simulink model "PVPanel"  (R2021b)
settings: Solver=FixedStepDiscrete  StartTime=0.0  StopTime=inf  RelTol=1e-3
PreLoadFcn:
  | %
  | Fc=3780;                          % PWM Carrier frequency (Hz)
  | Ts_Power=1/Fc/200;         % Simscape Power Systems sample time (s)
  | Ts_Control=20*Ts_Power;  % Inverter Control system sample time (s)
InitFcn:
  | %
  | Fc=3780;                          % PWM Carrier frequency (Hz)
  | Ts_Power=1/Fc/200;         % Simscape Power Systems sample time (s)
  | Ts_Control=20*Ts_Power;  % Inverter Control system sample time (s)
undefined symbols (not defined in the file): Acid, Lead
libraries: spsGroundLib x18, spsVoltageMeasurementLib x18, spsCurrentMeasurementLib x12, spsSeriesRLCBranchLib x10, spsParallelRLCBranchLib x6, spsBreakerLib x6, spsDiodeLib x6, spsBoostConverterLib x4, spsBatteryLib x2, spsPVArrayLib x2, spspowerguiLib x1
settings Model: Creator=MathWorks  LastModifiedBy=masangofi
settings SolverCC: AlgebraicLoopSolver=TrustRegion
settings DataIOCC: SaveFormat=Structure  SignalLoggingSaveFormat=ModelDataLogs  SaveOutput=off  SignalLogging=off  DSMLogging=off  SaveTime=off  ReturnWorkspaceOutputs=off
settings OptimizationCC: ExpressionDepthLimit=2147483647  LifeSpan=inf
settings DebuggingCC: UnderspecifiedInitializationDetection=Classic  MergeDetectMultiDrivingBlocksExec=none  SolverPrmCheckMsg=warning  FcnCallInpInsideContextMsg=warning  AllowSymbolicDim=off  StateNameClashWarn=warning  SFUnexpectedBacktrackingDiag=warning  SFNoUnconditionalDefaultTransitionDiag=warning  SFExecutionAtInitializationDiag=none  SFMachineParentedDataDiag=warning  ArithmeticOperatorsInVariantConditions=warning
settings HardwareCC: ProdBitPerPointer=32  ProdBitPerSizeT=32  ProdBitPerPtrDiffT=32  ProdLargestAtomicFloat=None  ProdIntDivRoundTo=Undefined  ProdEndianess=Unspecified  ProdWordSize=32  ProdHWDeviceType=32-bit Generic
settings ModelReferenceCC: PropagateSignalLabelsOutOfModel=off
settings SFSimCC: SimUseLocalCustomCode=off  CustomCodeUndefinedFunction=UseInterfaceOnly
settings RTWCC: RTWUseLocalCustomCode=off
settings CodeAppCC: StateflowObjectComments=on
settings GRTTargetCC: TargetLangStandard=C89/C90 (ANSI)  CombineOutputUpdateFcns=off  GRTInterface=on
settings ConfigComp: CovMetricSettings=dw  CovSaveCumulativeToWorkspaceVar=on  CovSaveSingleToWorkspaceVar=on  CovExternalEMLEnable=off  CovSFcnEnable=off
settings SimscapeCC: SimscapeNormalizeSystem=off

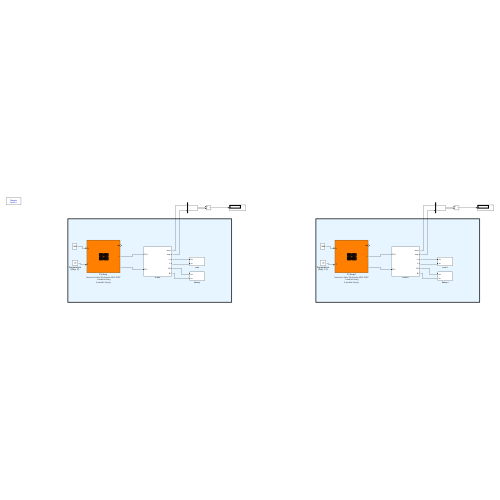
[thumbnail: Simulink's stored preview of the top-level diagram]
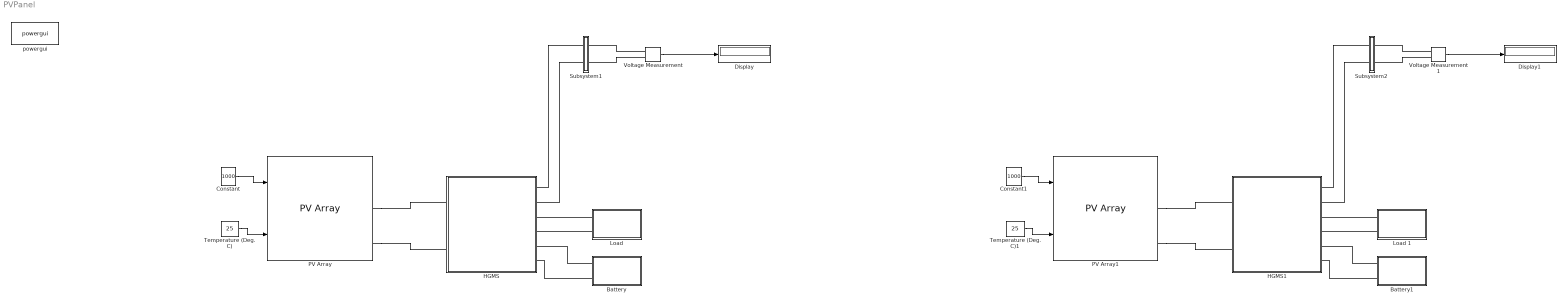
== system PVPanel ==
  Battery : Subsystem
  Battery1 : Subsystem
  Constant : Constant  Value=1000
  Constant1 : Constant  Value=1000
  Display : Display
  Display1 : Display
  HGMS : Subsystem
  HGMS1 : Subsystem
  "Load " : Subsystem
  Load 1 : Subsystem
  PV Array : spsPVArrayLib/PV Array  Npar=5  Nser=1  PlotType=one module @ 25 deg.C & specified irradiances  S_vec=[160 80 40 20 10 ]  Temp_C_vec=[ 4 ]  ModuleName=American Solar Wholesale ASW-220P  PlotWhenSelected=off  Pm=219.765  Ncell=60  Voc=36.24  Isc=7.77  Vm=29.9  Im=7.35  beta_Voc_pc=-0.33  alpha_Isc_pc=0.05  beta_Voc=-0.11959  alpha_Isc=0.003885  IL=7.8511  I0=8.7896e-11  nI=0.9332  Rsh=197.4106  Rs=0.27009  RobustModel=off  RobustCellTemperature=313.3991  BAL=on  Tc=1e-6  Tfilter=5e-5
      settings: AttributesFormatString=|
      | %<ModuleName>
      | %<Nser>-module string
      | %<Npar> parallel strings
  PV Array1 : spsPVArrayLib/PV Array  Npar=5  Nser=1  PlotType=one module @ 25 deg.C & specified irradiances  S_vec=[160 80 40 20 10 ]  Temp_C_vec=[ 4 ]  ModuleName=American Solar Wholesale ASW-220P  PlotWhenSelected=off  Pm=219.765  Ncell=60  Voc=36.24  Isc=7.77  Vm=29.9  Im=7.35  beta_Voc_pc=-0.33  alpha_Isc_pc=0.05  beta_Voc=-0.11959  alpha_Isc=0.003885  IL=7.8511  I0=8.7896e-11  nI=0.9332  Rsh=197.4106  Rs=0.27009  RobustModel=off  RobustCellTemperature=313.3991  BAL=on  Tc=1e-6  Tfilter=5e-5
      settings: AttributesFormatString=|
      | %<ModuleName>
      | %<Nser>-module string
      | %<Npar> parallel strings
  Subsystem1 : Subsystem
  Subsystem2 : Subsystem
  Temperature (Deg. C) : Constant  Value=25
  Temperature (Deg. C)1 : Constant  Value=25
  Voltage Measurement : spsVoltageMeasurementLib/Voltage Measurement  PhasorSimulation=off  OutputType=Complex  PSBequivalent=0
  Voltage Measurement1 : spsVoltageMeasurementLib/Voltage Measurement  PhasorSimulation=off  OutputType=Complex  PSBequivalent=0
  powergui : spspowerguiLib/powergui  Priority=1  SimulationMode=Discrete  SampleTime=50e-6  frequency=60  Iterations=50  frequencyindice=0  Pbase=100e6  ErrMax=1e-4  UnitsV=kV  UnitsW=MW  buscounter=0  FunctionMessages=off  echomessages=off  EnableUseOfTLC=off  CurrentSourceSwitches=off  DisableSnubberDevices=off  DisableRonSwitches=off  DisableVfSwitches=off  DisplayEquations=off  AutomaticDiscreteSolvers=off  SolverType=Tustin/Backward Euler (TBE)  Interpol=off  ExternalGateDelay=off  methode=off  Ts=100  x0status=blocks  SPID=on  SwTol=0  HookPort=off  NonlinearTolerance=1e-4  nMaxIteration=100  ContinueOnMaxIteration=off  RestoreLinks=warning  ResistiveCurrentMeasurement=off  Frange=[0:2:500]  Ylog=off  Xlog=on  ShowGrid=off  save=off  variable=ZData  structure=0  ZoomFFT=off  StartTime=0.0  cycles=1  DisplayStyle=1  fundamental=60  FreqAxis=off  MaxFrequency=1000  frequencyindicesteady=1  RmsSteady=1  display=off
  wires:
  Temperature (Deg. C)/1 -> PV Array/2
  Constant/1 -> PV Array/1
  Voltage Measurement/1 -> Display/1
  Voltage Measurement1/1 -> Display1/1
  Constant1/1 -> PV Array1/1
  Temperature (Deg. C)1/1 -> PV Array1/2
  connections:
  "Load "/LConn2 -- HGMS/RConn4
  Subsystem1/LConn2 -- HGMS/RConn2
  Subsystem1/LConn1 -- HGMS/RConn1
  Voltage Measurement/LConn1 -- Subsystem1/RConn1
  Voltage Measurement/LConn2 -- Subsystem1/RConn2
  Battery/LConn2 -- HGMS/RConn6
  Battery/LConn1 -- HGMS/RConn5
  "Load "/LConn1 -- HGMS/RConn3
  PV Array/RConn2 -- HGMS/LConn2
  PV Array/RConn1 -- HGMS/LConn1
  Voltage Measurement1/LConn1 -- Subsystem2/RConn1
  Load 1/LConn1 -- HGMS1/RConn3
  Load 1/LConn2 -- HGMS1/RConn4
  Subsystem2/LConn2 -- HGMS1/RConn2
  Subsystem2/LConn1 -- HGMS1/RConn1
  Battery1/LConn2 -- HGMS1/RConn6
  Battery1/LConn1 -- HGMS1/RConn5
  PV Array1/RConn1 -- HGMS1/LConn1
  PV Array1/RConn2 -- HGMS1/LConn2
  Voltage Measurement1/LConn2 -- Subsystem2/RConn2

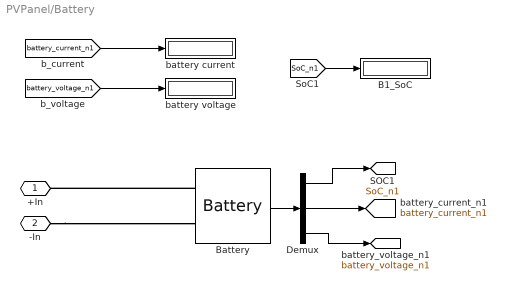
== system PVPanel/Battery ==
  B1_SoC : Display
  Battery : spsBatteryLib/Battery  BatType=Lead-Acid  ShowTempParam=off  ThermalPreset=no  ShowAgeParam=off  NomV=48  NomQ=70  SOC=70  Batt_Tr=1  PresetModel=on  MaxQ=72.9167  MinV=36  FullV=52.2632  Dis_rate=14  R=0.0068571  Normal_OP=21.7194  expZone="[48.8684     0.233333]"  current=[6.5 13 32.5]  Units=Time  Tci=20  NomT=20  T2=-30  MaxQ2=4.8  FullV2=7.1  Normal_OP2=5.655  expZone2="[6.58           1]"  Rca=0.6  ti=2000  Dp=0  Neq0=0  Tsim=1e6  Ta1=25  Qeol=5.4*0.9  Reol=0.013333*1.2  Char_age=[2.3478, 3]  Dis_age=[2.3478, 10]  N1=1500  N2=10500  N3=1000  N4=1400  Ta2=45  N5=950
  Demux : Demux  Outputs=3
  battery current : Display
  battery voltage : Display
  +In : PMIOPort  Side=Left
  -In : PMIOPort  Port=2  Side=Left
  tag scope: SoC_n1=global, battery_current_n1=global, battery_voltage_n1=global
  wires:
  Battery/1 -> Demux/1
  Demux/1 -> [SoC_n1]
  Demux/3 -> [battery_voltage_n1]
  Demux/2 -> [battery_current_n1]
  [SoC_n1] -> B1_SoC/1
  [battery_current_n1] -> battery current/1
  [battery_voltage_n1] -> battery voltage/1
  connections:
  -In/RConn1 -- Battery/LConn2
  Battery/LConn1 -- +In/RConn1

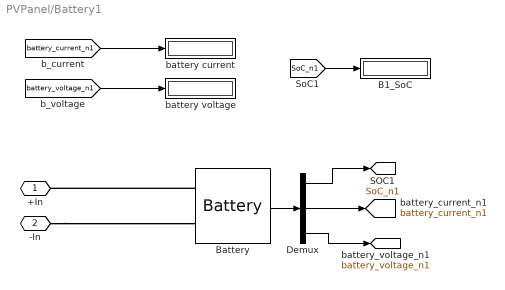
== system PVPanel/Battery1 ==
  B1_SoC : Display
  Battery : spsBatteryLib/Battery  BatType=Lead-Acid  ShowTempParam=off  ThermalPreset=no  ShowAgeParam=off  NomV=48  NomQ=70  SOC=70  Batt_Tr=1  PresetModel=on  MaxQ=72.9167  MinV=36  FullV=52.2632  Dis_rate=14  R=0.0068571  Normal_OP=21.7194  expZone="[48.8684     0.233333]"  current=[6.5 13 32.5]  Units=Time  Tci=20  NomT=20  T2=-30  MaxQ2=4.8  FullV2=7.1  Normal_OP2=5.655  expZone2="[6.58           1]"  Rca=0.6  ti=2000  Dp=0  Neq0=0  Tsim=1e6  Ta1=25  Qeol=5.4*0.9  Reol=0.013333*1.2  Char_age=[2.3478, 3]  Dis_age=[2.3478, 10]  N1=1500  N2=10500  N3=1000  N4=1400  Ta2=45  N5=950
  Demux : Demux  Outputs=3
  battery current : Display
  battery voltage : Display
  +In : PMIOPort  Side=Left
  -In : PMIOPort  Port=2  Side=Left
  tag scope: SoC_n1=global, battery_current_n1=global, battery_voltage_n1=global
  wires:
  Battery/1 -> Demux/1
  Demux/1 -> [SoC_n1]
  Demux/3 -> [battery_voltage_n1]
  Demux/2 -> [battery_current_n1]
  [SoC_n1] -> B1_SoC/1
  [battery_current_n1] -> battery current/1
  [battery_voltage_n1] -> battery voltage/1
  connections:
  -In/RConn1 -- Battery/LConn2
  Battery/LConn1 -- +In/RConn1

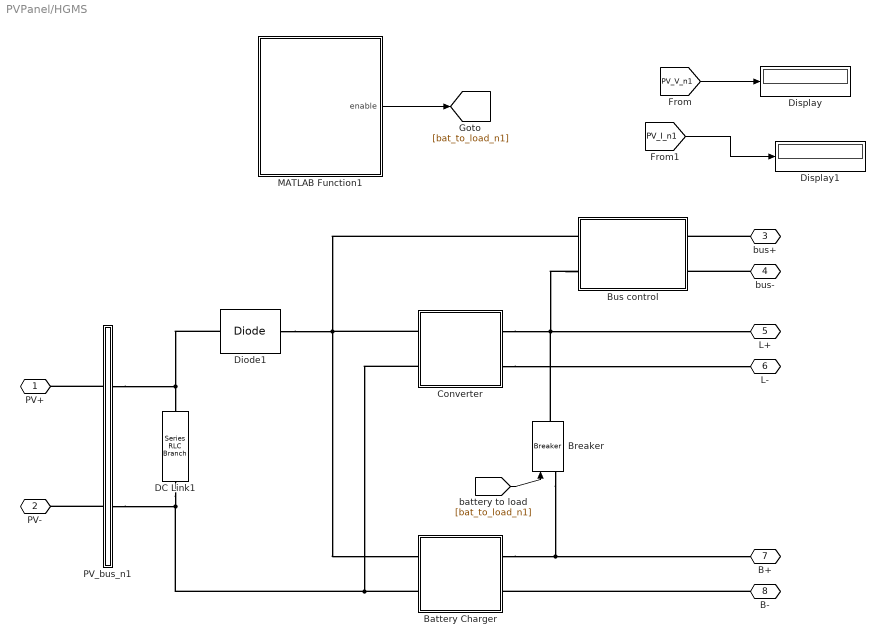
== system PVPanel/HGMS ==
  Battery Charger : Subsystem
  Breaker : spsBreakerLib/Breaker  InitialState=0  SwitchingTimes="[1/60  5/60]"  External=on  BreakerResistance=0.01  SnubberResistance=1e6  SnubberCapacitance=inf  Measurements=None  MoreParameters=on  NoBreakLoop=off
      settings: SourceProductBaseCode=PS
  Bus control : Subsystem
  Converter : Subsystem
  DC Link1 : spsSeriesRLCBranchLib/Series RLC Branch  LConnTagsString=__new0  RConnTagsString=__new0  BranchType=C  Resistance=1.0  Inductance=1.0  SetiL0=off  InitialCurrent=0  Capacitance=1000e-6  Setx0=off  InitialVoltage=48  Measurements=None
  Diode1 : spsDiodeLib/Diode  Ron=0.001  Lon=0  Vf=0.8  IC=0  UseSnubber=0  Rs=inf  Cs=250e-9  Measurements=off
  Display : Display
  Display1 : Display
  MATLAB Function1 : MATLAB Function  TreatAsAtomicUnit=on
  PV_bus_n1 : Subsystem
  PV+ : PMIOPort  Side=Left
  PV- : PMIOPort  Port=2  Side=Left
  bus+ : PMIOPort  Port=3  Side=Right
  bus- : PMIOPort  Port=4  Side=Right
  L+ : PMIOPort  Port=5  Side=Right
  L- : PMIOPort  Port=6  Side=Right
  B+ : PMIOPort  Port=7  Side=Right
  B- : PMIOPort  Port=8  Side=Right
  wires:
  MATLAB Function1/1(enable) -> [bat_to_load_n1]
  [bat_to_load_n1] -> Breaker/1
  [PV_V_n1] -> Display/1
  [PV_I_n1] -> Display1/1
  connections:
  Battery Charger/LConn2 -- Converter/LConn2 -- PV_bus_n1/RConn2 -- DC Link1/RConn1
  Converter/RConn1 -- Bus control/LConn2 -- Breaker/RConn1 -- L+/RConn1
  Converter/RConn2 -- L-/RConn1
  bus-/RConn1 -- Bus control/RConn2
  bus+/RConn1 -- Bus control/RConn1
  Battery Charger/RConn1 -- Breaker/LConn1 -- B+/RConn1
  B-/RConn1 -- Battery Charger/RConn2
  Diode1/RConn1 -- Bus control/LConn1 -- Converter/LConn1 -- Battery Charger/LConn1
  Diode1/LConn1 -- PV_bus_n1/RConn1 -- DC Link1/LConn1
  PV_bus_n1/LConn1 -- PV+/RConn1
  PV_bus_n1/LConn2 -- PV-/RConn1

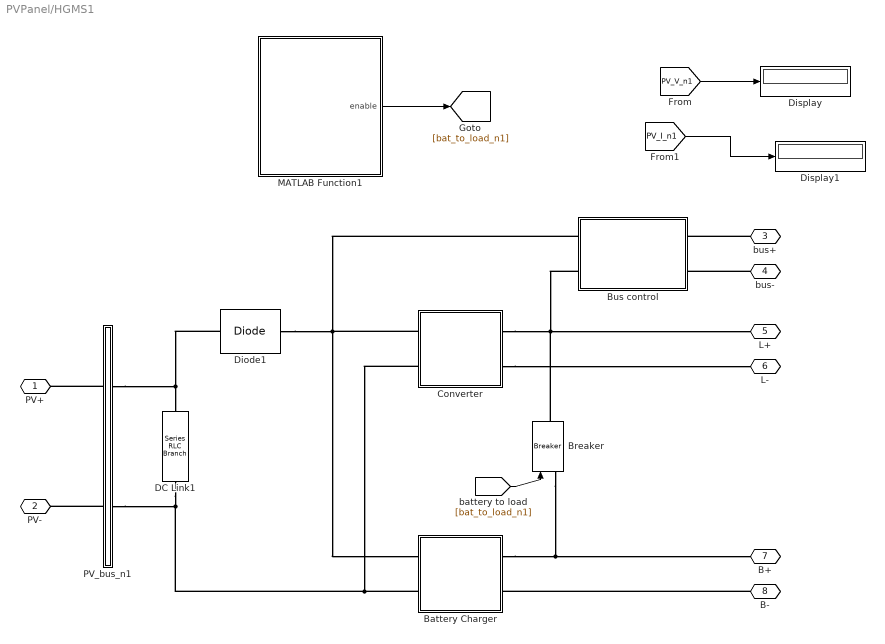
== system PVPanel/HGMS1 ==
  Battery Charger : Subsystem
  Breaker : spsBreakerLib/Breaker  InitialState=0  SwitchingTimes="[1/60  5/60]"  External=on  BreakerResistance=0.01  SnubberResistance=1e6  SnubberCapacitance=inf  Measurements=None  MoreParameters=on  NoBreakLoop=off
      settings: SourceProductBaseCode=PS
  Bus control : Subsystem
  Converter : Subsystem
  DC Link1 : spsSeriesRLCBranchLib/Series RLC Branch  LConnTagsString=__new0  RConnTagsString=__new0  BranchType=C  Resistance=1.0  Inductance=1.0  SetiL0=off  InitialCurrent=0  Capacitance=1000e-6  Setx0=off  InitialVoltage=48  Measurements=None
  Diode1 : spsDiodeLib/Diode  Ron=0.001  Lon=0  Vf=0.8  IC=0  UseSnubber=0  Rs=inf  Cs=250e-9  Measurements=off
  Display : Display
  Display1 : Display
  MATLAB Function1 : MATLAB Function  TreatAsAtomicUnit=on
  PV_bus_n1 : Subsystem
  PV+ : PMIOPort  Side=Left
  PV- : PMIOPort  Port=2  Side=Left
  bus+ : PMIOPort  Port=3  Side=Right
  bus- : PMIOPort  Port=4  Side=Right
  L+ : PMIOPort  Port=5  Side=Right
  L- : PMIOPort  Port=6  Side=Right
  B+ : PMIOPort  Port=7  Side=Right
  B- : PMIOPort  Port=8  Side=Right
  wires:
  MATLAB Function1/1(enable) -> [bat_to_load_n1]
  [bat_to_load_n1] -> Breaker/1
  [PV_V_n1] -> Display/1
  [PV_I_n1] -> Display1/1
  connections:
  Battery Charger/LConn2 -- PV_bus_n1/RConn2 -- DC Link1/RConn1 -- Converter/LConn2
  Converter/RConn1 -- Breaker/RConn1 -- L+/RConn1 -- Bus control/LConn2
  Converter/RConn2 -- L-/RConn1
  bus-/RConn1 -- Bus control/RConn2
  bus+/RConn1 -- Bus control/RConn1
  Battery Charger/RConn1 -- Breaker/LConn1 -- B+/RConn1
  B-/RConn1 -- Battery Charger/RConn2
  Converter/LConn1 -- Battery Charger/LConn1 -- Diode1/RConn1 -- Bus control/LConn1
  Diode1/LConn1 -- DC Link1/LConn1 -- PV_bus_n1/RConn1
  PV_bus_n1/LConn1 -- PV+/RConn1
  PV_bus_n1/LConn2 -- PV-/RConn1

== system PVPanel/Load  ==
  Parallel RLC Branch : spsParallelRLCBranchLib/Parallel RLC Branch  LConnTagsString=a  RConnTagsString=__new0  BranchType=R  Resistance=10000  Inductance=1e-3  SetiL0=off  InitialCurrent=0  Capacitance=1e-6  Setx0=off  InitialVoltage=0  Measurements=None
  +In : PMIOPort  Side=Left
  -In : PMIOPort  Port=2  Side=Left
  connections:
  Parallel RLC Branch/LConn1 -- +In/RConn1
  -In/RConn1 -- Parallel RLC Branch/RConn1

== system PVPanel/Load 1 ==
  Parallel RLC Branch : spsParallelRLCBranchLib/Parallel RLC Branch  LConnTagsString=a  RConnTagsString=__new0  BranchType=R  Resistance=10000  Inductance=1e-3  SetiL0=off  InitialCurrent=0  Capacitance=1e-6  Setx0=off  InitialVoltage=0  Measurements=None
  +In : PMIOPort  Side=Left
  -In : PMIOPort  Port=2  Side=Left
  connections:
  Parallel RLC Branch/LConn1 -- +In/RConn1
  -In/RConn1 -- Parallel RLC Branch/RConn1

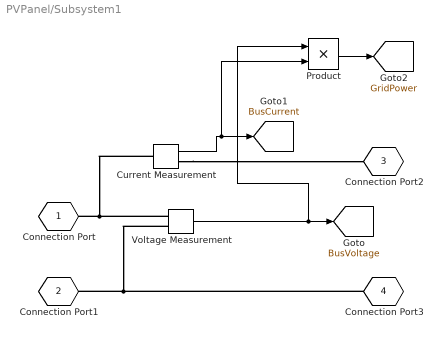
== system PVPanel/Subsystem1 ==
  Current Measurement : spsCurrentMeasurementLib/Current Measurement  PhasorSimulation=off  OutputType=Complex  PSBequivalent=0
  Product : Product
  Voltage Measurement : spsVoltageMeasurementLib/Voltage Measurement  PhasorSimulation=off  OutputType=Complex  PSBequivalent=0
  Connection Port : PMIOPort  Tag=PMCPort  Side=Left
  Connection Port1 : PMIOPort  Tag=PMCPort  Port=2  Side=Left
  Connection Port2 : PMIOPort  Tag=PMCPort  Port=3  Side=Right
  Connection Port3 : PMIOPort  Tag=PMCPort  Port=4  Side=Right
  tag scope: BusCurrent=global, BusVoltage=global, GridPower=global
  wires:
  Current Measurement/1 -> Product/2, [BusCurrent]
  Voltage Measurement/1 -> Product/1, [BusVoltage]
  Product/1 -> [GridPower]
  connections:
  Current Measurement/LConn1 -- Voltage Measurement/LConn1 -- Connection Port/RConn1
  Current Measurement/RConn1 -- Connection Port2/RConn1
  Voltage Measurement/LConn2 -- Connection Port3/RConn1 -- Connection Port1/RConn1

== system PVPanel/Subsystem2 ==
  Current Measurement : spsCurrentMeasurementLib/Current Measurement  PhasorSimulation=off  OutputType=Complex  PSBequivalent=0
  Product : Product
  Voltage Measurement : spsVoltageMeasurementLib/Voltage Measurement  PhasorSimulation=off  OutputType=Complex  PSBequivalent=0
  Connection Port : PMIOPort  Tag=PMCPort  Side=Left
  Connection Port1 : PMIOPort  Tag=PMCPort  Port=2  Side=Left
  Connection Port2 : PMIOPort  Tag=PMCPort  Port=3  Side=Right
  Connection Port3 : PMIOPort  Tag=PMCPort  Port=4  Side=Right
  tag scope: BusCurrent=global, BusVoltage=global, GridPower=global
  wires:
  Current Measurement/1 -> Product/2, [BusCurrent]
  Voltage Measurement/1 -> Product/1, [BusVoltage]
  Product/1 -> [GridPower]
  connections:
  Current Measurement/LConn1 -- Voltage Measurement/LConn1 -- Connection Port/RConn1
  Current Measurement/RConn1 -- Connection Port2/RConn1
  Voltage Measurement/LConn2 -- Connection Port3/RConn1 -- Connection Port1/RConn1

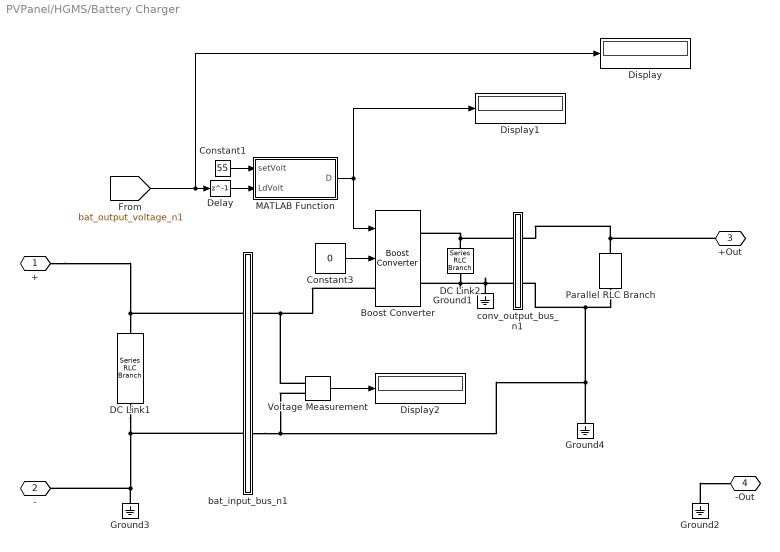
== system PVPanel/HGMS/Battery Charger ==
  Boost Converter : spsBoostConverterLib/Boost Converter  ModelType=Average model (D-controlled)  Ron=1e-6  Rs=1e6  Cs=inf  Vforward=[0,0]  Ron_Diode=1e-3  Rs_Diode=1e6  Cs_Diode=inf  Vf_Diode=1e-3  Rs_CurrentSource=1e6
      settings: SourceProductBaseCode=PS
  Constant1 : Constant  Value=55  OutDataTypeStr=double
  Constant3 : Constant  Value=0
  DC Link1 : spsSeriesRLCBranchLib/Series RLC Branch  LConnTagsString=__new0  RConnTagsString=__new0  BranchType=C  Resistance=1.0  Inductance=1.0  SetiL0=off  InitialCurrent=0  Capacitance=1000e-6  Setx0=off  InitialVoltage=0  Measurements=None
  DC Link2 : spsSeriesRLCBranchLib/Series RLC Branch  LConnTagsString=__new0  RConnTagsString=__new0  BranchType=C  Resistance=1.0  Inductance=1.0  SetiL0=off  InitialCurrent=0  Capacitance=100e-6  Setx0=off  InitialVoltage=0  Measurements=None
  Delay : Delay  DelayLength=1  InitialCondition=0
  Display : Display
  Display1 : Display
  Display2 : Display
  Ground{1..4} (4 alike) : spsGroundLib/Ground  LConnTagsString=a
  MATLAB Function : MATLAB Function  TreatAsAtomicUnit=on
  Parallel RLC Branch : spsParallelRLCBranchLib/Parallel RLC Branch  LConnTagsString=a  RConnTagsString=__new0  BranchType=R  Resistance=10e3  Inductance=1e-3  SetiL0=off  InitialCurrent=0  Capacitance=1e-6  Setx0=off  InitialVoltage=0  Measurements=None
  Voltage Measurement : spsVoltageMeasurementLib/Voltage Measurement  PhasorSimulation=off  OutputType=Complex  PSBequivalent=0
  bat_input_bus_n1 : Subsystem
  conv_output_bus_n1 : Subsystem
  + : PMIOPort  Side=Left
  - : PMIOPort  Port=2  Side=Left
  +Out : PMIOPort  Port=3  Side=Right
  -Out : PMIOPort  Port=4  Side=Right
  wires:
  Delay/1 -> MATLAB Function/2(LdVolt)
  [bat_output_voltage_n1] -> Display/1, Delay/1
  Constant3/1 -> Boost Converter/2
  Constant1/1 -> MATLAB Function/1(setVolt)
  MATLAB Function/1(D) -> Boost Converter/1, Display1/1
  Voltage Measurement/1 -> Display2/1
  connections:
  +/RConn1 -- DC Link1/LConn1 -- bat_input_bus_n1/LConn1
  DC Link1/RConn1 -- Ground3/LConn1 -- -/RConn1 -- bat_input_bus_n1/LConn2
  Boost Converter/RConn2 -- DC Link2/RConn1 -- conv_output_bus_n1/LConn2 -- Ground1/LConn1
  DC Link2/LConn1 -- Boost Converter/RConn1 -- conv_output_bus_n1/LConn1
  Ground4/LConn1 -- Voltage Measurement/LConn2 -- bat_input_bus_n1/RConn2 -- conv_output_bus_n1/RConn2 -- Parallel RLC Branch/RConn1
  Parallel RLC Branch/LConn1 -- conv_output_bus_n1/RConn1 -- +Out/RConn1
  Boost Converter/LConn1 -- Voltage Measurement/LConn1 -- bat_input_bus_n1/RConn1
  Ground2/LConn1 -- -Out/RConn1

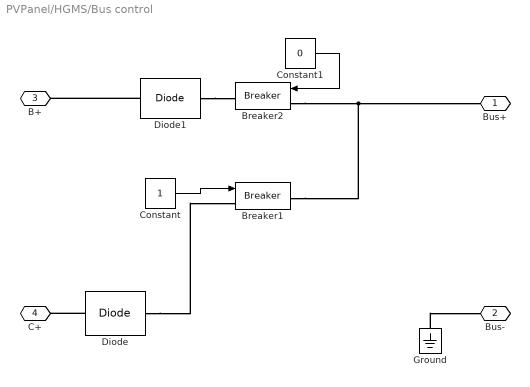
== system PVPanel/HGMS/Bus control ==
  Breaker1 : spsBreakerLib/Breaker  InitialState=0  SwitchingTimes="[1/60  5/60]"  External=on  BreakerResistance=0.01  SnubberResistance=1e6  SnubberCapacitance=inf  Measurements=None  MoreParameters=on  NoBreakLoop=off
      settings: SourceProductBaseCode=PS
  Breaker2 : spsBreakerLib/Breaker  InitialState=0  SwitchingTimes="[1/60  5/60]"  External=on  BreakerResistance=0.01  SnubberResistance=1e6  SnubberCapacitance=inf  Measurements=None  MoreParameters=on  NoBreakLoop=off
      settings: SourceProductBaseCode=PS
  Constant : Constant
  Constant1 : Constant  Value=0
  Diode : spsDiodeLib/Diode  Ron=0.001  Lon=0  Vf=0.8  IC=0  UseSnubber=0  Rs=500  Cs=250e-9  Measurements=off
  Diode1 : spsDiodeLib/Diode  Ron=0.001  Lon=0  Vf=0.8  IC=0  UseSnubber=0  Rs=500  Cs=250e-9  Measurements=off
  Ground : spsGroundLib/Ground  LConnTagsString=a
  Bus+ : PMIOPort  Side=Right
  Bus- : PMIOPort  Port=2  Side=Right
  B+ : PMIOPort  Port=3  Side=Left
  C+ : PMIOPort  Port=4  Side=Left
  wires:
  Constant/1 -> Breaker1/1
  Constant1/1 -> Breaker2/1
  connections:
  Breaker1/RConn1 -- Breaker2/LConn1 -- Bus+/RConn1
  Ground/LConn1 -- Bus-/RConn1
  Diode/LConn1 -- C+/RConn1
  Diode/RConn1 -- Breaker1/LConn1
  Diode1/RConn1 -- B+/RConn1
  Diode1/LConn1 -- Breaker2/RConn1

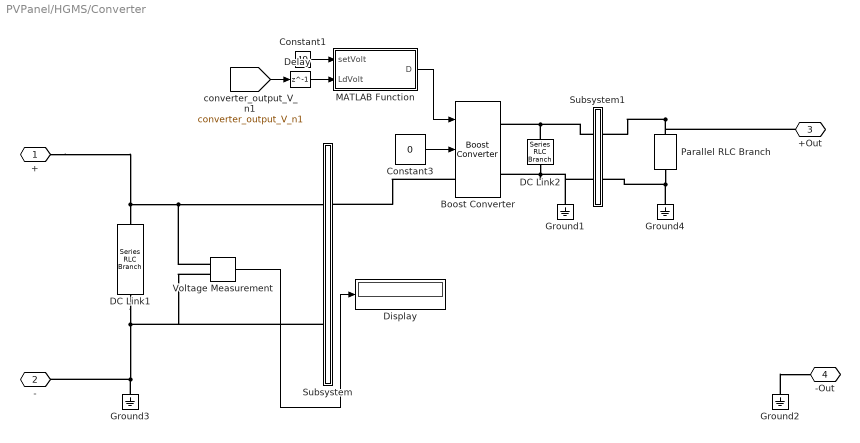
== system PVPanel/HGMS/Converter ==
  Boost Converter : spsBoostConverterLib/Boost Converter  ModelType=Average model (D-controlled)  Ron=1e-6  Rs=1e6  Cs=inf  Vforward=[0,0]  Ron_Diode=1e-3  Rs_Diode=1e6  Cs_Diode=inf  Vf_Diode=1e-3  Rs_CurrentSource=inf
      settings: SourceProductBaseCode=PS
  Constant1 : Constant  Value=49  OutDataTypeStr=double
  Constant3 : Constant  Value=0
  DC Link1 : spsSeriesRLCBranchLib/Series RLC Branch  LConnTagsString=__new0  RConnTagsString=__new0  BranchType=C  Resistance=1.0  Inductance=1.0  SetiL0=off  InitialCurrent=0  Capacitance=1000e-6  Setx0=off  InitialVoltage=0  Measurements=None
  DC Link2 : spsSeriesRLCBranchLib/Series RLC Branch  LConnTagsString=__new0  RConnTagsString=__new0  BranchType=C  Resistance=1.0  Inductance=1.0  SetiL0=off  InitialCurrent=0  Capacitance=100e-6  Setx0=off  InitialVoltage=0  Measurements=None
  Delay : Delay  DelayLength=1  InitialCondition=0
  Display : Display
  Ground{1..4} (4 alike) : spsGroundLib/Ground  LConnTagsString=a
  MATLAB Function : MATLAB Function  TreatAsAtomicUnit=on
  Parallel RLC Branch : spsParallelRLCBranchLib/Parallel RLC Branch  LConnTagsString=a  RConnTagsString=__new0  BranchType=R  Resistance=10e3  Inductance=1e-3  SetiL0=off  InitialCurrent=0  Capacitance=1e-6  Setx0=off  InitialVoltage=0  Measurements=None
  Subsystem : Subsystem
  Subsystem1 : Subsystem
  Voltage Measurement : spsVoltageMeasurementLib/Voltage Measurement  PhasorSimulation=off  OutputType=Complex  PSBequivalent=0
  + : PMIOPort  Side=Left
  - : PMIOPort  Port=2  Side=Left
  +Out : PMIOPort  Port=3  Side=Right
  -Out : PMIOPort  Port=4  Side=Right
  wires:
  Delay/1 -> MATLAB Function/2(LdVolt)
  [converter_output_V_n1] -> Delay/1
  Constant3/1 -> Boost Converter/2
  Constant1/1 -> MATLAB Function/1(setVolt)
  MATLAB Function/1(D) -> Boost Converter/1
  Voltage Measurement/1 -> Display/1
  connections:
  +/RConn1 -- Voltage Measurement/LConn1 -- Subsystem/LConn1 -- DC Link1/LConn1
  DC Link1/RConn1 -- Voltage Measurement/LConn2 -- Subsystem/LConn2 -- Ground3/LConn1 -- -/RConn1
  DC Link2/RConn1 -- Subsystem1/LConn2 -- Ground1/LConn1 -- Boost Converter/RConn2
  DC Link2/LConn1 -- Subsystem1/LConn1 -- Boost Converter/RConn1
  Parallel RLC Branch/RConn1 -- Subsystem1/RConn2 -- Ground4/LConn1
  Boost Converter/LConn1 -- Subsystem/RConn1
  Ground2/LConn1 -- -Out/RConn1
  Parallel RLC Branch/LConn1 -- Subsystem1/RConn1 -- +Out/RConn1

== system PVPanel/HGMS/PV_bus_n1 ==
  Current Measurement : spsCurrentMeasurementLib/Current Measurement  PhasorSimulation=off  OutputType=Complex  PSBequivalent=0
  Voltage Measurement : spsVoltageMeasurementLib/Voltage Measurement  PhasorSimulation=off  OutputType=Complex  PSBequivalent=0
  Connection Port : PMIOPort  Tag=PMCPort  Side=Left
  Connection Port1 : PMIOPort  Tag=PMCPort  Port=2  Side=Left
  Connection Port2 : PMIOPort  Tag=PMCPort  Port=3  Side=Right
  Connection Port3 : PMIOPort  Tag=PMCPort  Port=4  Side=Right
  tag scope: PV_I_n1=global, PV_V_n1=global
  wires:
  Current Measurement/1 -> [PV_I_n1]
  Voltage Measurement/1 -> [PV_V_n1]
  connections:
  Current Measurement/LConn1 -- Voltage Measurement/LConn1 -- Connection Port/RConn1
  Current Measurement/RConn1 -- Connection Port2/RConn1
  Voltage Measurement/LConn2 -- Connection Port3/RConn1 -- Connection Port1/RConn1

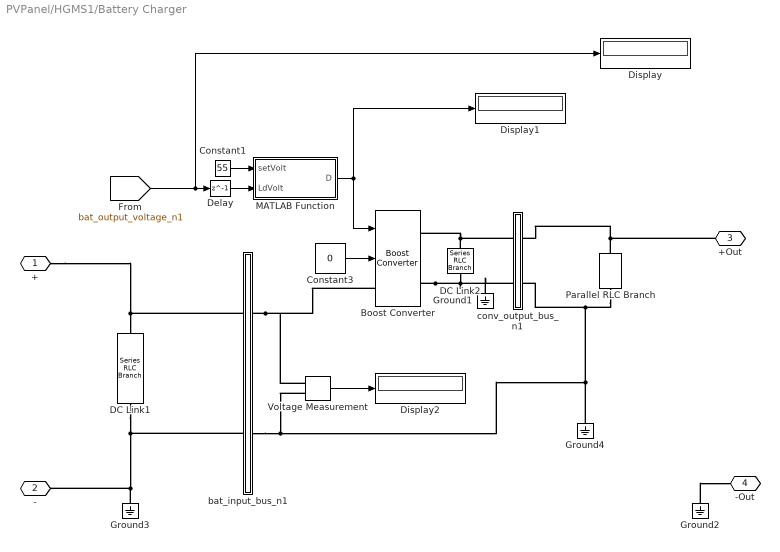
== system PVPanel/HGMS1/Battery Charger ==
  Boost Converter : spsBoostConverterLib/Boost Converter  ModelType=Average model (D-controlled)  Ron=1e-6  Rs=1e6  Cs=inf  Vforward=[0,0]  Ron_Diode=1e-3  Rs_Diode=1e6  Cs_Diode=inf  Vf_Diode=1e-3  Rs_CurrentSource=1e6
      settings: SourceProductBaseCode=PS
  Constant1 : Constant  Value=55  OutDataTypeStr=double
  Constant3 : Constant  Value=0
  DC Link1 : spsSeriesRLCBranchLib/Series RLC Branch  LConnTagsString=__new0  RConnTagsString=__new0  BranchType=C  Resistance=1.0  Inductance=1.0  SetiL0=off  InitialCurrent=0  Capacitance=1000e-6  Setx0=off  InitialVoltage=0  Measurements=None
  DC Link2 : spsSeriesRLCBranchLib/Series RLC Branch  LConnTagsString=__new0  RConnTagsString=__new0  BranchType=C  Resistance=1.0  Inductance=1.0  SetiL0=off  InitialCurrent=0  Capacitance=100e-6  Setx0=off  InitialVoltage=0  Measurements=None
  Delay : Delay  DelayLength=1  InitialCondition=0
  Display : Display
  Display1 : Display
  Display2 : Display
  Ground{1..4} (4 alike) : spsGroundLib/Ground  LConnTagsString=a
  MATLAB Function : MATLAB Function  TreatAsAtomicUnit=on
  Parallel RLC Branch : spsParallelRLCBranchLib/Parallel RLC Branch  LConnTagsString=a  RConnTagsString=__new0  BranchType=R  Resistance=10e3  Inductance=1e-3  SetiL0=off  InitialCurrent=0  Capacitance=1e-6  Setx0=off  InitialVoltage=0  Measurements=None
  Voltage Measurement : spsVoltageMeasurementLib/Voltage Measurement  PhasorSimulation=off  OutputType=Complex  PSBequivalent=0
  bat_input_bus_n1 : Subsystem
  conv_output_bus_n1 : Subsystem
  + : PMIOPort  Side=Left
  - : PMIOPort  Port=2  Side=Left
  +Out : PMIOPort  Port=3  Side=Right
  -Out : PMIOPort  Port=4  Side=Right
  wires:
  Delay/1 -> MATLAB Function/2(LdVolt)
  [bat_output_voltage_n1] -> Display/1, Delay/1
  Constant3/1 -> Boost Converter/2
  Constant1/1 -> MATLAB Function/1(setVolt)
  MATLAB Function/1(D) -> Boost Converter/1, Display1/1
  Voltage Measurement/1 -> Display2/1
  connections:
  +/RConn1 -- DC Link1/LConn1 -- bat_input_bus_n1/LConn1
  DC Link1/RConn1 -- Ground3/LConn1 -- -/RConn1 -- bat_input_bus_n1/LConn2
  Boost Converter/RConn2 -- DC Link2/RConn1 -- conv_output_bus_n1/LConn2 -- Ground1/LConn1
  DC Link2/LConn1 -- Boost Converter/RConn1 -- conv_output_bus_n1/LConn1
  Voltage Measurement/LConn2 -- bat_input_bus_n1/RConn2 -- Ground4/LConn1 -- Parallel RLC Branch/RConn1 -- conv_output_bus_n1/RConn2
  +Out/RConn1 -- Parallel RLC Branch/LConn1 -- conv_output_bus_n1/RConn1
  bat_input_bus_n1/RConn1 -- Boost Converter/LConn1 -- Voltage Measurement/LConn1
  Ground2/LConn1 -- -Out/RConn1

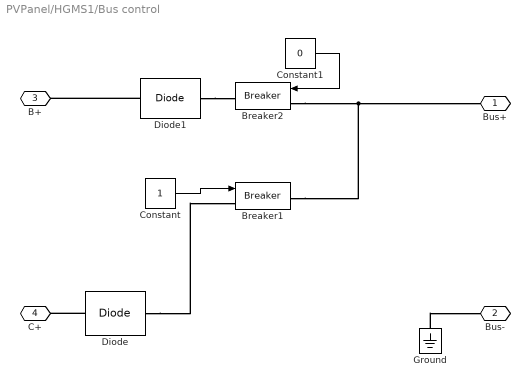
== system PVPanel/HGMS1/Bus control ==
  Breaker1 : spsBreakerLib/Breaker  InitialState=0  SwitchingTimes="[1/60  5/60]"  External=on  BreakerResistance=0.01  SnubberResistance=1e6  SnubberCapacitance=inf  Measurements=None  MoreParameters=on  NoBreakLoop=off
      settings: SourceProductBaseCode=PS
  Breaker2 : spsBreakerLib/Breaker  InitialState=0  SwitchingTimes="[1/60  5/60]"  External=on  BreakerResistance=0.01  SnubberResistance=1e6  SnubberCapacitance=inf  Measurements=None  MoreParameters=on  NoBreakLoop=off
      settings: SourceProductBaseCode=PS
  Constant : Constant
  Constant1 : Constant  Value=0
  Diode : spsDiodeLib/Diode  Ron=0.001  Lon=0  Vf=0.8  IC=0  UseSnubber=0  Rs=500  Cs=250e-9  Measurements=off
  Diode1 : spsDiodeLib/Diode  Ron=0.001  Lon=0  Vf=0.8  IC=0  UseSnubber=0  Rs=500  Cs=250e-9  Measurements=off
  Ground : spsGroundLib/Ground  LConnTagsString=a
  Bus+ : PMIOPort  Side=Right
  Bus- : PMIOPort  Port=2  Side=Right
  B+ : PMIOPort  Port=3  Side=Left
  C+ : PMIOPort  Port=4  Side=Left
  wires:
  Constant/1 -> Breaker1/1
  Constant1/1 -> Breaker2/1
  connections:
  Breaker1/RConn1 -- Bus+/RConn1 -- Breaker2/LConn1
  Ground/LConn1 -- Bus-/RConn1
  Diode/LConn1 -- C+/RConn1
  Diode/RConn1 -- Breaker1/LConn1
  Diode1/RConn1 -- B+/RConn1
  Diode1/LConn1 -- Breaker2/RConn1

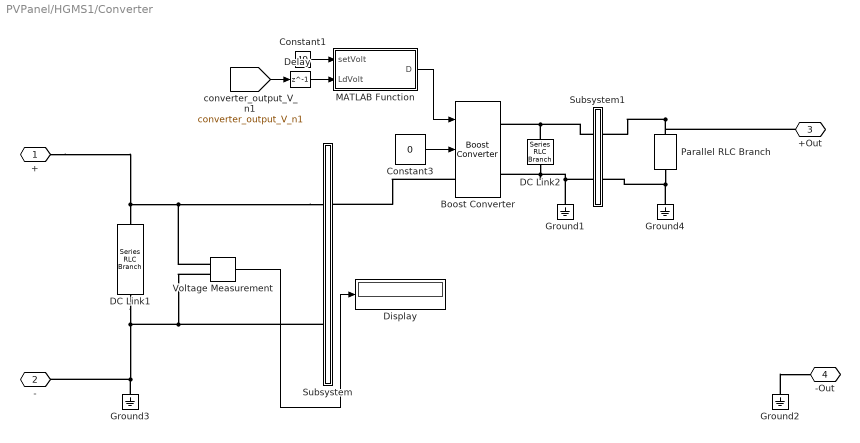
== system PVPanel/HGMS1/Converter ==
  Boost Converter : spsBoostConverterLib/Boost Converter  ModelType=Average model (D-controlled)  Ron=1e-6  Rs=1e6  Cs=inf  Vforward=[0,0]  Ron_Diode=1e-3  Rs_Diode=1e6  Cs_Diode=inf  Vf_Diode=1e-3  Rs_CurrentSource=inf
      settings: SourceProductBaseCode=PS
  Constant1 : Constant  Value=49  OutDataTypeStr=double
  Constant3 : Constant  Value=0
  DC Link1 : spsSeriesRLCBranchLib/Series RLC Branch  LConnTagsString=__new0  RConnTagsString=__new0  BranchType=C  Resistance=1.0  Inductance=1.0  SetiL0=off  InitialCurrent=0  Capacitance=1000e-6  Setx0=off  InitialVoltage=0  Measurements=None
  DC Link2 : spsSeriesRLCBranchLib/Series RLC Branch  LConnTagsString=__new0  RConnTagsString=__new0  BranchType=C  Resistance=1.0  Inductance=1.0  SetiL0=off  InitialCurrent=0  Capacitance=100e-6  Setx0=off  InitialVoltage=0  Measurements=None
  Delay : Delay  DelayLength=1  InitialCondition=0
  Display : Display
  Ground{1..4} (4 alike) : spsGroundLib/Ground  LConnTagsString=a
  MATLAB Function : MATLAB Function  TreatAsAtomicUnit=on
  Parallel RLC Branch : spsParallelRLCBranchLib/Parallel RLC Branch  LConnTagsString=a  RConnTagsString=__new0  BranchType=R  Resistance=10e3  Inductance=1e-3  SetiL0=off  InitialCurrent=0  Capacitance=1e-6  Setx0=off  InitialVoltage=0  Measurements=None
  Subsystem : Subsystem
  Subsystem1 : Subsystem
  Voltage Measurement : spsVoltageMeasurementLib/Voltage Measurement  PhasorSimulation=off  OutputType=Complex  PSBequivalent=0
  + : PMIOPort  Side=Left
  - : PMIOPort  Port=2  Side=Left
  +Out : PMIOPort  Port=3  Side=Right
  -Out : PMIOPort  Port=4  Side=Right
  wires:
  Delay/1 -> MATLAB Function/2(LdVolt)
  [converter_output_V_n1] -> Delay/1
  Constant3/1 -> Boost Converter/2
  Constant1/1 -> MATLAB Function/1(setVolt)
  MATLAB Function/1(D) -> Boost Converter/1
  Voltage Measurement/1 -> Display/1
  connections:
  Subsystem/LConn1 -- +/RConn1 -- DC Link1/LConn1 -- Voltage Measurement/LConn1
  DC Link1/RConn1 -- Ground3/LConn1 -- -/RConn1 -- Subsystem/LConn2 -- Voltage Measurement/LConn2
  DC Link2/RConn1 -- Boost Converter/RConn2 -- Subsystem1/LConn2 -- Ground1/LConn1
  Boost Converter/RConn1 -- DC Link2/LConn1 -- Subsystem1/LConn1
  Parallel RLC Branch/RConn1 -- Ground4/LConn1 -- Subsystem1/RConn2
  Boost Converter/LConn1 -- Subsystem/RConn1
  Ground2/LConn1 -- -Out/RConn1
  +Out/RConn1 -- Parallel RLC Branch/LConn1 -- Subsystem1/RConn1

== system PVPanel/HGMS1/PV_bus_n1 ==
  Current Measurement : spsCurrentMeasurementLib/Current Measurement  PhasorSimulation=off  OutputType=Complex  PSBequivalent=0
  Voltage Measurement : spsVoltageMeasurementLib/Voltage Measurement  PhasorSimulation=off  OutputType=Complex  PSBequivalent=0
  Connection Port : PMIOPort  Tag=PMCPort  Side=Left
  Connection Port1 : PMIOPort  Tag=PMCPort  Port=2  Side=Left
  Connection Port2 : PMIOPort  Tag=PMCPort  Port=3  Side=Right
  Connection Port3 : PMIOPort  Tag=PMCPort  Port=4  Side=Right
  tag scope: PV_I_n1=global, PV_V_n1=global
  wires:
  Current Measurement/1 -> [PV_I_n1]
  Voltage Measurement/1 -> [PV_V_n1]
  connections:
  Current Measurement/LConn1 -- Voltage Measurement/LConn1 -- Connection Port/RConn1
  Current Measurement/RConn1 -- Connection Port2/RConn1
  Voltage Measurement/LConn2 -- Connection Port3/RConn1 -- Connection Port1/RConn1

== system PVPanel/HGMS/Battery Charger/bat_input_bus_n1 ==
  Current Measurement : spsCurrentMeasurementLib/Current Measurement  PhasorSimulation=off  OutputType=Complex  PSBequivalent=0
  Voltage Measurement : spsVoltageMeasurementLib/Voltage Measurement  PhasorSimulation=off  OutputType=Complex  PSBequivalent=0
  Connection Port : PMIOPort  Tag=PMCPort  Side=Left
  Connection Port1 : PMIOPort  Tag=PMCPort  Port=2  Side=Left
  Connection Port2 : PMIOPort  Tag=PMCPort  Port=3  Side=Right
  Connection Port3 : PMIOPort  Tag=PMCPort  Port=4  Side=Right
  tag scope: Source_voltage_n1=global, source_current_n1=global
  wires:
  Current Measurement/1 -> [source_current_n1]
  Voltage Measurement/1 -> [Source_voltage_n1]
  connections:
  Current Measurement/LConn1 -- Connection Port/RConn1 -- Voltage Measurement/LConn1
  Current Measurement/RConn1 -- Connection Port2/RConn1
  Voltage Measurement/LConn2 -- Connection Port3/RConn1 -- Connection Port1/RConn1

== system PVPanel/HGMS/Battery Charger/conv_output_bus_n1 ==
  Current Measurement : spsCurrentMeasurementLib/Current Measurement  PhasorSimulation=off  OutputType=Complex  PSBequivalent=0
  Voltage Measurement : spsVoltageMeasurementLib/Voltage Measurement  PhasorSimulation=off  OutputType=Complex  PSBequivalent=0
  Connection Port : PMIOPort  Tag=PMCPort  Side=Left
  Connection Port1 : PMIOPort  Tag=PMCPort  Port=2  Side=Left
  Connection Port2 : PMIOPort  Tag=PMCPort  Port=3  Side=Right
  Connection Port3 : PMIOPort  Tag=PMCPort  Port=4  Side=Right
  tag scope: bat_output_current_n1=global, bat_output_voltage_n1=global
  wires:
  Current Measurement/1 -> [bat_output_current_n1]
  Voltage Measurement/1 -> [bat_output_voltage_n1]
  connections:
  Current Measurement/LConn1 -- Voltage Measurement/LConn1 -- Connection Port/RConn1
  Current Measurement/RConn1 -- Connection Port2/RConn1
  Voltage Measurement/LConn2 -- Connection Port3/RConn1 -- Connection Port1/RConn1

== system PVPanel/HGMS/Converter/Subsystem ==
  Current Measurement : spsCurrentMeasurementLib/Current Measurement  PhasorSimulation=off  OutputType=Complex  PSBequivalent=0
  Voltage Measurement : spsVoltageMeasurementLib/Voltage Measurement  PhasorSimulation=off  OutputType=Complex  PSBequivalent=0
  Connection Port : PMIOPort  Tag=PMCPort  Side=Left
  Connection Port1 : PMIOPort  Tag=PMCPort  Port=2  Side=Left
  Connection Port2 : PMIOPort  Tag=PMCPort  Port=3  Side=Right
  Connection Port3 : PMIOPort  Tag=PMCPort  Port=4  Side=Right
  tag scope: converter_input_I_n1=global, converter_input_V_n1=global
  wires:
  Current Measurement/1 -> [converter_input_I_n1]
  Voltage Measurement/1 -> [converter_input_V_n1]
  connections:
  Current Measurement/LConn1 -- Voltage Measurement/LConn1 -- Connection Port/RConn1
  Current Measurement/RConn1 -- Connection Port2/RConn1
  Voltage Measurement/LConn2 -- Connection Port3/RConn1 -- Connection Port1/RConn1

== system PVPanel/HGMS/Converter/Subsystem1 ==
  Current Measurement1 : spsCurrentMeasurementLib/Current Measurement  PhasorSimulation=off  OutputType=Complex  PSBequivalent=0
  Voltage Measurement1 : spsVoltageMeasurementLib/Voltage Measurement  PhasorSimulation=off  OutputType=Complex  PSBequivalent=0
  Connection Port4 : PMIOPort  Tag=PMCPort  Side=Left
  Connection Port5 : PMIOPort  Tag=PMCPort  Port=2  Side=Left
  Connection Port6 : PMIOPort  Tag=PMCPort  Port=3  Side=Right
  Connection Port7 : PMIOPort  Tag=PMCPort  Port=4  Side=Right
  tag scope: converter_output_I_n1=global, converter_output_V_n1=global
  wires:
  Current Measurement1/1 -> [converter_output_I_n1]
  Voltage Measurement1/1 -> [converter_output_V_n1]
  connections:
  Connection Port5/RConn1 -- Voltage Measurement1/LConn2 -- Connection Port7/RConn1
  Connection Port4/RConn1 -- Current Measurement1/LConn1 -- Voltage Measurement1/LConn1
  Current Measurement1/RConn1 -- Connection Port6/RConn1

== system PVPanel/HGMS1/Battery Charger/bat_input_bus_n1 ==
  Current Measurement : spsCurrentMeasurementLib/Current Measurement  PhasorSimulation=off  OutputType=Complex  PSBequivalent=0
  Voltage Measurement : spsVoltageMeasurementLib/Voltage Measurement  PhasorSimulation=off  OutputType=Complex  PSBequivalent=0
  Connection Port : PMIOPort  Tag=PMCPort  Side=Left
  Connection Port1 : PMIOPort  Tag=PMCPort  Port=2  Side=Left
  Connection Port2 : PMIOPort  Tag=PMCPort  Port=3  Side=Right
  Connection Port3 : PMIOPort  Tag=PMCPort  Port=4  Side=Right
  tag scope: Source_voltage_n1=global, source_current_n1=global
  wires:
  Current Measurement/1 -> [source_current_n1]
  Voltage Measurement/1 -> [Source_voltage_n1]
  connections:
  Current Measurement/LConn1 -- Voltage Measurement/LConn1 -- Connection Port/RConn1
  Current Measurement/RConn1 -- Connection Port2/RConn1
  Voltage Measurement/LConn2 -- Connection Port3/RConn1 -- Connection Port1/RConn1

== system PVPanel/HGMS1/Battery Charger/conv_output_bus_n1 ==
  Current Measurement : spsCurrentMeasurementLib/Current Measurement  PhasorSimulation=off  OutputType=Complex  PSBequivalent=0
  Voltage Measurement : spsVoltageMeasurementLib/Voltage Measurement  PhasorSimulation=off  OutputType=Complex  PSBequivalent=0
  Connection Port : PMIOPort  Tag=PMCPort  Side=Left
  Connection Port1 : PMIOPort  Tag=PMCPort  Port=2  Side=Left
  Connection Port2 : PMIOPort  Tag=PMCPort  Port=3  Side=Right
  Connection Port3 : PMIOPort  Tag=PMCPort  Port=4  Side=Right
  tag scope: bat_output_current_n1=global, bat_output_voltage_n1=global
  wires:
  Current Measurement/1 -> [bat_output_current_n1]
  Voltage Measurement/1 -> [bat_output_voltage_n1]
  connections:
  Current Measurement/LConn1 -- Voltage Measurement/LConn1 -- Connection Port/RConn1
  Current Measurement/RConn1 -- Connection Port2/RConn1
  Voltage Measurement/LConn2 -- Connection Port3/RConn1 -- Connection Port1/RConn1

== system PVPanel/HGMS1/Converter/Subsystem ==
  Current Measurement : spsCurrentMeasurementLib/Current Measurement  PhasorSimulation=off  OutputType=Complex  PSBequivalent=0
  Voltage Measurement : spsVoltageMeasurementLib/Voltage Measurement  PhasorSimulation=off  OutputType=Complex  PSBequivalent=0
  Connection Port : PMIOPort  Tag=PMCPort  Side=Left
  Connection Port1 : PMIOPort  Tag=PMCPort  Port=2  Side=Left
  Connection Port2 : PMIOPort  Tag=PMCPort  Port=3  Side=Right
  Connection Port3 : PMIOPort  Tag=PMCPort  Port=4  Side=Right
  tag scope: converter_input_I_n1=global, converter_input_V_n1=global
  wires:
  Current Measurement/1 -> [converter_input_I_n1]
  Voltage Measurement/1 -> [converter_input_V_n1]
  connections:
  Current Measurement/LConn1 -- Voltage Measurement/LConn1 -- Connection Port/RConn1
  Current Measurement/RConn1 -- Connection Port2/RConn1
  Voltage Measurement/LConn2 -- Connection Port3/RConn1 -- Connection Port1/RConn1

== system PVPanel/HGMS1/Converter/Subsystem1 ==
  Current Measurement1 : spsCurrentMeasurementLib/Current Measurement  PhasorSimulation=off  OutputType=Complex  PSBequivalent=0
  Voltage Measurement1 : spsVoltageMeasurementLib/Voltage Measurement  PhasorSimulation=off  OutputType=Complex  PSBequivalent=0
  Connection Port4 : PMIOPort  Tag=PMCPort  Side=Left
  Connection Port5 : PMIOPort  Tag=PMCPort  Port=2  Side=Left
  Connection Port6 : PMIOPort  Tag=PMCPort  Port=3  Side=Right
  Connection Port7 : PMIOPort  Tag=PMCPort  Port=4  Side=Right
  tag scope: converter_output_I_n1=global, converter_output_V_n1=global
  wires:
  Current Measurement1/1 -> [converter_output_I_n1]
  Voltage Measurement1/1 -> [converter_output_V_n1]
  connections:
  Connection Port7/RConn1 -- Connection Port5/RConn1 -- Voltage Measurement1/LConn2
  Voltage Measurement1/LConn1 -- Connection Port4/RConn1 -- Current Measurement1/LConn1
  Current Measurement1/RConn1 -- Connection Port6/RConn1

== matlab function PVPanel/HGMS/Converter/MATLAB Function ==
  data: setVolt input; LdVolt input; D output
function D = fcn(setVolt, LdVolt)

persistent Duty;
persistent DutyLim;
persistent change;


if isempty(DutyLim)
    DutyLim = 0.85;
end

if LdVolt < 8
    DutyLim = 0.10;
end

if LdVolt < setVolt - 8
    if DutyLim == 0.10
        DutyLim = 0.85;
    end
end

if isempty(Duty)
    Duty = 0.10;
end

if setVolt < LdVolt
    Duty = Duty-0.001;
    if Duty <=0
        Duty=0;
    end
end

if setVolt > LdVolt
    Duty = Duty+0.0001;
    if Duty >DutyLim
        Duty = DutyLim;
    end
end


D=Duty;
end

== matlab function PVPanel/HGMS/Battery Charger/MATLAB Function ==
  data: setVolt input; LdVolt input; D output
function D = fcn(setVolt, LdVolt)

persistent Duty;
persistent DutyLim;
persistent change;


if isempty(DutyLim)
    DutyLim = 0.90;
end

if LdVolt < 8
    DutyLim = 0.10;
end

if LdVolt < setVolt - 8
    if DutyLim == 0.10
        DutyLim = 0.90;
    end
end

if isempty(Duty)
    Duty = 0.10;
end

if setVolt < LdVolt
    Duty = Duty-0.001;
    if Duty <=0
        Duty=0;
    end
end

if setVolt > LdVolt
    Duty = Duty+0.0001;
    if Duty >DutyLim
        Duty = DutyLim;
    end
end


D=Duty;
end

== matlab function PVPanel/HGMS1/Battery Charger/MATLAB Function ==
  data: setVolt input; LdVolt input; D output
function D = fcn(setVolt, LdVolt)

persistent Duty;
persistent DutyLim;
persistent change;


if isempty(DutyLim)
    DutyLim = 0.90;
end

if LdVolt < 8
    DutyLim = 0.10;
end

if LdVolt < setVolt - 8
    if DutyLim == 0.10
        DutyLim = 0.90;
    end
end

if isempty(Duty)
    Duty = 0.10;
end

if setVolt < LdVolt
    Duty = Duty-0.001;
    if Duty <=0
        Duty=0;
    end
end

if setVolt > LdVolt
    Duty = Duty+0.0001;
    if Duty >DutyLim
        Duty = DutyLim;
    end
end


D=Duty;
end

== matlab function PVPanel/HGMS/MATLAB Function1 ==
  data: enable output
function enable   = fcn

enable = 0;

== matlab function PVPanel/HGMS1/Converter/MATLAB Function ==
  data: setVolt input; LdVolt input; D output
function D = fcn(setVolt, LdVolt)

persistent Duty;
persistent DutyLim;
persistent change;


if isempty(DutyLim)
    DutyLim = 0.85;
end

if LdVolt < 8
    DutyLim = 0.10;
end

if LdVolt < setVolt - 8
    if DutyLim == 0.10
        DutyLim = 0.85;
    end
end

if isempty(Duty)
    Duty = 0.10;
end

if setVolt < LdVolt
    Duty = Duty-0.001;
    if Duty <=0
        Duty=0;
    end
end

if setVolt > LdVolt
    Duty = Duty+0.0001;
    if Duty >DutyLim
        Duty = DutyLim;
    end
end


D=Duty;
end

== matlab function PVPanel/HGMS1/MATLAB Function1 ==
  data: enable output
function enable   = fcn

enable = 0;
